simulink library "hose_pump_unit_v4"  (R2025b)
settings: Solver=VariableStepAuto  StartTime=0.0  StopTime=10.0  RelTol=1e-3
undefined symbols (not defined in the file): ACV_fit_coeffs, HP_bladder_elastic_modulus, HP_flowrate_damping_coefficient, HP_unstretched_fiber_angle, HP_unstretched_length, HP_unstretched_radius, HP_unstretched_wall_thickness, L_inlet, mu, power_avg_start_time, PTO_capacity_W, R_inlet, regulator_set_pressure_PSI, simu, SV_closing_threshold_Pa, SV_opening_threshold_Pa, turbine_gear_ratio
libraries: simulink x28, dspstat3 x4, turbine_generator_v0 x2, dsppolyfun x1, adjustable_check_valve_v0 x1
(part 2 of 2)

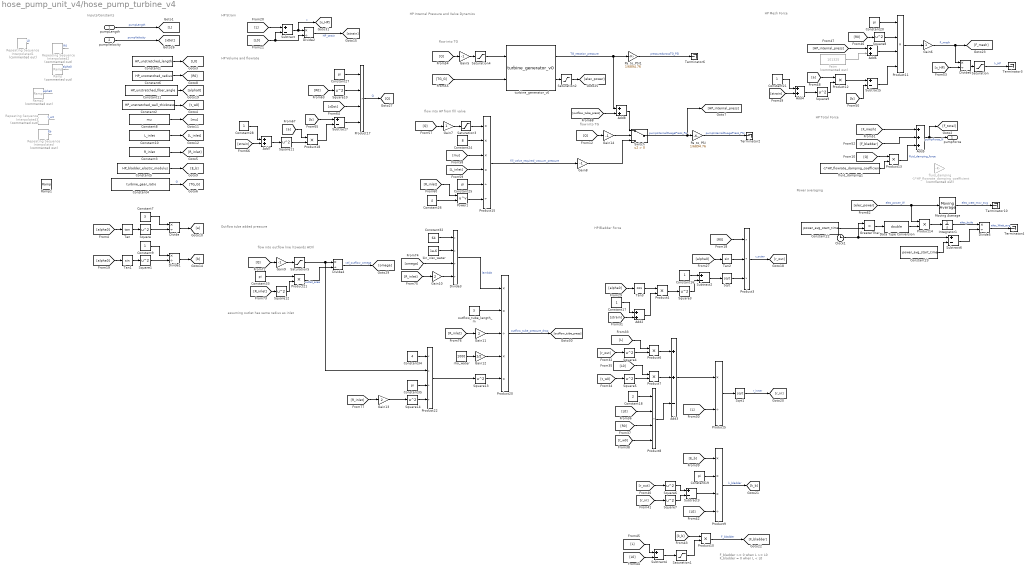
== system hose_pump_unit_v4/hose_pump_turbine_v4 ==
  note: Power averaging
  note: Outflow tube added pressure
  note: assuming outlet has same radius as inlet
  note: flow into outflow line (towards ACV)
  note: flow into HP from fill valve
  note: Inputs/Constants
  note: HP Volume and flowrate
  note: HP Strain
  note: HP Internal Pressure and Valve Dynamics
  note: HP Bladder Force
  note: HP Mesh Force
  note: HP Total Force
  note: F_bladder >= 0 when L >= L0
      | F_bladder = 0 when L < L0
  note: flow into TG
  note: flow into TG
  pumpLength : Inport
  pumpVelocity : Inport  Port=2
  Add{2,4,6..8} (5 alike) : Sum
  Add3 : Sum  Inputs=++-
  Add5 : Sum  Inputs=+++
  Clock1 : Clock
  Constant1 : Constant  Value=HP_unstretched_length
  Constant10 : Constant  Value=L_inlet
  Constant11 : Constant  Value=HP_unstretched_fiber_angle
  Constant{9,16..17,21,28} (5 alike) : Constant
  Constant18 : Constant  Value=2
  Constant{19..20,25,27,33,35} (6 alike) : Constant  Value=pi
  Constant2 : Constant  Value=HP_unstretched_wall_thickness
  Constant22 : Constant  Value=power_avg_start_time
  Constant23 : Constant  Value=power_avg_start_time
  Constant24 : Constant  Value=8
  Constant26 : Constant  Value=4
  Constant3 : Constant  Value=R_inlet
  Constant32 : Constant  Value=64
  Constant34 : Constant  Value=4
  Constant4 : Constant  Value=turbine_gear_ratio
  Constant5 : Constant  Value=HP_bladder_elastic_modulus
  Constant6 : Constant  Value=HP_unstretched_radius
  Constant7 : Constant  Value=3
  Constant8 : Constant  Value=mu
  Data Type Conversion : DataTypeConversion  OutDataTypeStr=double  SaturateOnIntegerOverflow=off  RndMeth=Floor
  Divide{,1..2,4..6} (6 alike) : Product  Inputs=*/
  Divide3 : Product  Inputs=**//
  Gain10 : Gain  Gain=2
  Gain11 : Gain  Gain=2
  Gain12 : Gain  Gain=1/2
  Gain13 : Gain  Gain=2
  Gain{5,8..9,14} (4 alike) : Gain  Gain=-1
  Gain6 : Gain
  Gain7 : Gain
  GreaterThan : RelationalOperator  Operator=>  OutDataTypeStr=boolean  RndMeth=Simplest  InputSameDT=off
  Integrator1 : Integrator
  Moving Average : dspstat3/Moving Average  Method=Sliding window  ForgettingFactorPort=off  SpecifyWindowLength=on  WindowLength=30 / simu.dt  OverlapLength=30 / simu.dt - 1  AllowArbitraryInputLength=off  ForgettingFactor=0.9  SimulateUsing=Interpreted execution
  Pa_to_PSI : Gain  Gain=1/6894.76
  Pa_to_PSI1 : Gain  Gain=1/6894.76
  Patm : Constant  Commented=on  Value=101325
  Power1 : Math  Operator=pow
  Product{4,6..7,10,12..14,18,21} (9 alike) : Product
  Product11 : Product  Inputs=****
  Product15 : Product  Inputs=****//
  Product17 : Product  Inputs=****
  Product20 : Product  Inputs=**/**
  Product22 : Product  Inputs=**//
  Product3 : Product  Inputs=*/*
  Product5 : Product  Inputs=*/
  Product8 : Product  Inputs=****
  Product9 : Product  Inputs=***/
  Ramp : simulink/Sources/Ramp  Commented=on  slope=(1.25-1.12) / 2400  start=30  InitialOutput=1.12
  Ramp1 : simulink/Sources/Ramp  slope=5/1200  start=30  InitialOutput=1
  Ramp2 : simulink/Sources/Ramp  Commented=on  slope=(1.1 - 0.9) * HP_unstretched_fiber_angle / 2400  start=30  InitialOutput=0.9 * HP_unstretched_fiber_angle
  Repeating Sequence Interpolated : simulink/Sources/Repeating Sequence Interpolated  Commented=on  OutValues=HP_bladder_elastic_modulus * [0.75 2 0.75]  TimeValues=[0 60 120]*2  LookUpMeth=Interpolation-Use End Values  tsamp=simu.dt  OutMin=[]  OutMax=[]  OutDataTypeStr=double  OutputDataTypeScalingMode=double  OutDataType=fixdt(0,8)  OutScaling=2^-10
  Repeating Sequence Interpolated1 : simulink/Sources/Repeating Sequence Interpolated  Commented=on  OutValues=HP_unstretched_length * [0.8 1.2 0.8]  TimeValues=[0 60 120] * 4  LookUpMeth=Interpolation-Use End Values  tsamp=simu.dt  OutMin=[]  OutMax=[]  OutDataTypeStr=double  OutputDataTypeScalingMode=double  OutDataType=fixdt(0,8)  OutScaling=2^-10
  Repeating Sequence Interpolated2 : simulink/Sources/Repeating Sequence Interpolated  Commented=on  OutValues=HP_unstretched_radius * [0.8 1.2 0.8]  TimeValues=[0 60 120] * 4  LookUpMeth=Interpolation-Use End Values  tsamp=simu.dt  OutMin=[]  OutMax=[]  OutDataTypeStr=double  OutputDataTypeScalingMode=double  OutDataType=fixdt(0,8)  OutScaling=2^-10
  Repeating Sequence Interpolated3 : simulink/Sources/Repeating Sequence Interpolated  Commented=on  OutValues=HP_unstretched_wall_thickness * [0.75 1.25 0.75]  TimeValues=[0 60 120] * 4  LookUpMeth=Interpolation-Use End Values  tsamp=simu.dt  OutMin=[]  OutMax=[]  OutDataTypeStr=double  OutputDataTypeScalingMode=double  OutDataType=fixdt(0,8)  OutScaling=2^-10
  Saturation : Saturate  UpperLimit=10000  LowerLimit=-10000
  Saturation1 : Saturate  UpperLimit=inf  LowerLimit=0
  Saturation2 : Saturate  UpperLimit=PTO_capacity_W  LowerLimit=-inf
  Saturation3 : Saturate  UpperLimit=inf  LowerLimit=0
  Saturation4 : Saturate  UpperLimit=inf  LowerLimit=0
  Saturation5 : Saturate  UpperLimit=inf  LowerLimit=1e-8
  Sqrt : Sqrt
  Sqrt1 : Sqrt
  Square{,1,3..14} (14 alike) : Math  Operator=square
  Subtract{,2..7} (7 alike) : Sum  Inputs=+-
  Switch : Switch  Criteria=u2 > Threshold  SaturateOnIntegerOverflow=off  InputSameDT=off
  Tan : Trigonometry  Operator=tan
  Tan1 : Trigonometry
  Tan2 : Trigonometry
  Tan3 : Trigonometry  Operator=cos
  Terminator{2..4,6,10} (5 alike) : Terminator
  fluid_damping : Gain  Commented=on  Gain=-1*HP_flowrate_damping_coefficient
  fluid_damping1 : Constant  Value=-1*HP_flowrate_damping_coefficient
  kin_visc_water : Constant  Value=1e-6
  outflow_tube_length_m : Constant  Value=3
  rho_water : Constant  Value=1000
  turbine_generator_v0 : turbine_generator_v0/turbine_generator_v0  SystemSampleTime=-1  VariantActivationTime=update diagram  EmptyChoice=off  PassThrough=off  PassThroughVariantControl=(default)  EmptyChoiceVariantControl=(default)  AllowFlexibleInterface=on  Latency=0  AutoFrameSizeCalculation=off
  pumpForce : Outport
  wires:
  Saturation2/1 -> [elec_power]
  Moving Average/1 -> Terminator10/1  "elec_watt_mov_avg"
  Product11/1 -> Gain6/1
  Ramp2/1 -> ?  "alpha0"
  fluid_damping1/1 -> Product13/2
  [Q] -> Product13/1
  Repeating Sequence Interpolated3/1 -> ?  "t_w0"
  Repeating Sequence Interpolated2/1 -> ?  "R0"
  Repeating Sequence Interpolated1/1 -> ?  "L0"
  Repeating Sequence Interpolated/1 -> ?  "Eb"
  Ramp/1 -> ?  "alpha0"
  Pa_to_PSI1/1 -> Terminator6/1  "pressureAcrossTG_PSI"
  Divide6/1 -> Saturation/1
  Saturation/1 -> Terminator3/1  "k_HP"
  [x_HP] -> Divide6/2
  Constant32/1 -> Divide3/1
  Constant33/1 -> Product21/1
  Gain9/1 -> Saturation5/1
  Gain11/1 -> Product20/3
  outflow_tube_length_m/1 -> Product20/2
  Square12/1 -> Product21/2
  [omega] -> Divide3/3
  Gain12/1 -> Product20/4
  Product21/1 -> Divide4/2  "outlet_area"
  Gain13/1 -> Square14/1
  [R_inlet] -> Gain10/1
  [R_inlet] -> Square12/1
  [R_inlet] -> Gain11/1
  Product22/1 -> Square13/1
  Square13/1 -> Product20/5
  Gain10/1 -> Divide3/4
  Divide4/1 -> [omega]  "vel_outflow_omega"
  kin_visc_water/1 -> Divide3/2
  [Q] -> Gain9/1
  Square14/1 -> Product22/4
  Constant35/1 -> Product22/3
  rho_water/1 -> Gain12/1
  Divide3/1 -> Product20/1  "lambda"
  Saturation5/1 -> Divide4/1, Product22/2
  Product20/1 -> [outflow_tube_press]  "outflow_tube_pressure_drop"
  Constant34/1 -> Product22/1
  [R_inlet] -> Gain13/1
  Add8/1 -> Switch/1
  Gain5/1 -> Saturation4/1
  Gain14/1 -> Switch/2
  Square11/1 -> Product18/2
  [a] -> Product18/1
  Add7/1 -> Square11/1
  Constant28/1 -> Add7/1
  [strain] -> Add7/2
  Product18/1 -> Subtract7/2
  [b] -> Subtract7/1
  Subtract7/1 -> Product17/4
  [xDot] -> Product17/3
  [R0] -> Square10/1
  Constant27/1 -> Product17/1
  Square10/1 -> Product17/2
  Product17/1 -> [Q]  "Q"
  pumpVelocity/1 -> [xDot]  "pumpVelocity"
  [F_bladder] -> Add5/2
  [F_mesh] -> Add5/1
  turbine_generator_v0/2 -> Saturation2/1
  Saturation4/1 -> turbine_generator_v0/1
  Gain8/1 -> Switch/3
  Product15/1 -> Gain8/1  "fill_valve_required_vacuum_pressure"
  Constant26/1 -> Power1/2
  [R_inlet] -> Power1/1
  Power1/1 -> Product15/6
  Constant25/1 -> Product15/5
  [L_inlet] -> Product15/4
  [mu] -> Product15/3
  Constant24/1 -> Product15/2
  Saturation3/1 -> Product15/1
  Gain7/1 -> Saturation3/1
  [Q] -> Gain7/1
  turbine_generator_v0/1 -> Add8/1, Pa_to_PSI1/1  "TG_reaction_pressure"
  [TG_G] -> turbine_generator_v0/2
  [Q] -> Gain5/1
  Saturation1/1 -> Product10/2
  Clock1/1 -> Subtract6/1, GreaterThan/1
  Data Type Conversion/1 -> Product14/2
  Constant22/1 -> GreaterThan/2
  Constant23/1 -> Subtract6/2
  Product14/1 -> Integrator1/1
  Subtract6/1 -> Divide5/2
  GreaterThan/1 -> Data Type Conversion/1
  Divide5/1 -> Terminator4/1  "elec_Watt_avg"
  Integrator1/1 -> Divide5/1  "elec_Joule"
  [elec_power] -> Product14/1, Moving Average/1  "elec_power_W"
  Add6/1 -> Product11/3
  Patm/1 -> Add6/2
  Add5/1 -> pumpForce/1, [F_total]  "pumpForce_N"
  Product13/1 -> Add5/3  "fluid_damping_force"
  Gain6/1 -> [F_mesh], Divide6/1  "F_mesh"
  Subtract5/1 -> Product11/4
  [b] -> Subtract5/2
  Product12/1 -> Subtract5/1
  Square9/1 -> Product12/2
  [strain] -> Add4/2
  Add4/1 -> Square9/1
  Constant21/1 -> Add4/1
  [a] -> Product12/1
  [HP_internal_press] -> Add6/1
  Square8/1 -> Product11/2
  Constant20/1 -> Product11/1
  [R0] -> Square8/1
  Product10/1 -> [F_bladder]  "F_bladder"
  [L] -> Subtract4/1
  [L0] -> Subtract4/2
  Subtract4/1 -> Saturation1/1
  [k_b] -> Product10/1
  Product9/1 -> [k_b]  "k_bladder"
  [L0] -> Product9/4
  Square7/1 -> Subtract3/2
  [r_in] -> Square7/1
  Square6/1 -> Subtract3/1
  [r_out] -> Square6/1
  Subtract3/1 -> Product9/3
  Constant19/1 -> Product9/2
  [E_b] -> Product9/1
  [t_w0] -> Product8/4
  [R0] -> Product8/3
  [L0] -> Product8/2
  Constant18/1 -> Product8/1
  Product8/1 -> Add3/3
  Product7/1 -> Add3/2
  Square5/1 -> Product7/2
  [t_w0] -> Square5/1
  [L0] -> Product7/1
  [L] -> Product6/1
  [r_out] -> Square4/1
  Square4/1 -> Product6/2
  Product6/1 -> Add3/1
  Add3/1 -> Product5/1
  [L] -> Product5/2
  Product5/1 -> Sqrt1/1
  Sqrt1/1 -> [r_in]  "r_inner"
  Product3/1 -> [r_out]  "r_outer"
  Add2/1 -> Product4/2
  [strain] -> Add2/2
  Constant17/1 -> Add2/1
  Tan3/1 -> Product4/1
  Product4/1 -> Square3/1
  Square3/1 -> Subtract2/2
  [alpha0] -> Tan3/1
  Constant16/1 -> Subtract2/1
  Subtract2/1 -> Sqrt/1
  Sqrt/1 -> Product3/3
  Tan2/1 -> Product3/2
  [alpha0] -> Tan2/1
  [R0] -> Product3/1
  Divide2/1 -> [strain]  "HP_strain"
  Subtract/1 -> Divide2/1, [x_HP]  "x"
  [L0] -> Subtract/2, Divide2/2
  [L] -> Subtract/1
  Constant9/1 -> Divide1/1
  [alpha0] -> Tan1/1
  Tan1/1 -> Square1/1
  Square1/1 -> Divide1/2
  Divide1/1 -> [b]
  Divide/1 -> [a]
  Square/1 -> Divide/2
  Tan/1 -> Square/1
  [alpha0] -> Tan/1
  Constant7/1 -> Divide/1
  Constant3/1 -> [R_inlet]
  Constant4/1 -> [TG_G]  "G"
  Pa_to_PSI/1 -> Terminator2/1  "pumpInternalGuagePress_PSI"
  Switch/1 -> Pa_to_PSI/1, [HP_internal_press]  "pumpInternalGuagePress_Pa"
  Constant10/1 -> [L_inlet]
  Constant8/1 -> [mu]
  Constant6/1 -> [R0]
  pumpLength/1 -> [L]  "pumpLength"
  Constant11/1 -> [alpha0]
  Constant5/1 -> [E_b]
  Constant1/1 -> [L0]
  Constant2/1 -> [t_w0]
  [outflow_tube_press] -> Add8/2
  [Q] -> Gain14/1

== stateflow chart hose_pump_unit_v4/hose_pump_accumulator_servo_valve_v4/Chart ==
  state valve_closed
    en:
    servo_valve_cmd = 0;
  state valve_opened
    en, du:
    servo_valve_cmd = 1;
  (default) -> valve_closed
  valve_closed -> valve_opened : [accumulator_press > opening_threshold_press]
  valve_opened -> valve_closed : [accumulator_press < closing_threshold_press]
  data: accumulator_press input size=1; opening_threshold_press input size=1; closing_threshold_press input size=1; servo_valve_cmd output size=1

== stateflow chart hose_pump_unit_v4/hose_pump_ACV_v4/Chart ==
  state wait
    en:
    zeroCrossing_prev = t;
    en, du:
    pumpedWater_internal = pumpedWater_internal + Q * dt;
  state update
    en:
    pumpWindowLength_sec = t - zeroCrossing_prev;
    pumpedWater_mL = pumpedWater_internal*1e3;
    pumpedWater_internal = 0;
  (default) -> update
  update -> wait : [Q ~= 0]
  wait -> update : [Q == 0]
  data: Q input; pumpWindowLength_sec output; zeroCrossing_prev local =0; pumpedWater_mL output =0; pumpedWater_internal local =0; dt local =simu.dt

== matlab function hose_pump_unit_v4/hose_pump_ACV_v4/MATLAB Function ==
  data: pumpDisp input; pumpVel input; CV_setting input; Qout output; r0 input; L0 input; alpha0 input; k_tube input; mu input; lt input; rt input; Qin output; F output; P input
function [Qout, Qin, F] = pumpDisplacementCalcs(pumpDisp, pumpVel, CV_setting, r0, L0, alpha0, k_tube, mu, lt, rt, P)

persistent a b
if isempty(a) % only need to calc these once
    a = 3/tan(alpha0)^2;
    b = 1/sin(alpha0)^2;
end

if pumpVel > 0 % pumping water out
    % P = CV_setting; % assume internal pressure immediately rises to check valve set pressure
    % F = pi * ru^2 * P * (3 * (pumpDisp/lu+1)^2 / (tan(au))^2 - 1/sin(au)^2) + k_tube*pumpDisp;
    Qout = -pi * ru^2 * (1/sin(alpha0)^2 - 3 * (pumpDisp/L0+1)^2 / (tan(alpha0))^2) * pumpVel;
    Qin = 0;
else
    % F = k_tube*pumpDisp;
    Qin = pi * ru^2 * (1/sin(alpha0)^2 - 3 * (pumpDisp/L0+1)^2 / (tan(alpha0))^2) * pumpVel;
    Qout = 0;
    % P = -8*mu*lt/(pi*rt^4)*Qin;
end

F = pi * ru^2 * max([P, 0]) * (3 * (pumpDisp/L0+1)^2 / (tan(alpha0))^2 - 1/sin(alpha0)^2) + k_tube*pumpDisp;

== matlab function hose_pump_unit_v4/hose_pump_ACV_v4/pumpInternalPressure ==
  data: CV_setting input; mu input; lt input; rt input; Q input; P output
function P  = pumpInternalPressure(CV_setting, mu, lt, rt, Q)
% Patm = 101325; %Pa
if Q < 0 % pumping water out
    P = CV_setting;
    %debug = [8*mu*lt/(pi*rt^4)*Qout, CV_setting];
else
    P = -8*mu*lt/(pi*rt^4)*Q;
end
